simulink model "lab3_teil3fcn"  (R2018b)
settings: Solver=ode23t  StartTime=0.0  StopTime=10.0  RelTol=1e-12  AbsTol=1e-12
values from neighbouring files (symbols this model uses):
  AK = pi/4 * dK^2    (= 0.000314159265359)    [lab3_teil2.m]    (also in lab3_teil3.m; modelbildung_lab3.m)
  dB = 2.8e-3    (= 0.0028)    [lab3_teil2.m]    (also in lab3_teil3.m; modelbildung_lab3.m)
  FR = 5    [lab3_teil2.m]    (also in lab3_teil3.m; modelbildung_lab3.m)
  m = 1    [lab3_teil2.m]    (also in lab3_teil3.m; modelbildung_lab3.m)
  nB = table(:,2)    [lab3_teil3.m]
  rho = 850    [lab3_teil2.m]    (also in lab3_teil3.m; modelbildung_lab3.m)
  xB = table(:,1)    [lab3_teil3.m]
  zeta = 0.5    [lab3_teil2.m]    (also in lab3_teil3.m; modelbildung_lab3.m)
libraries: simulink x1
settings Model: Creator=Naveen  LastModifiedBy=Naveen

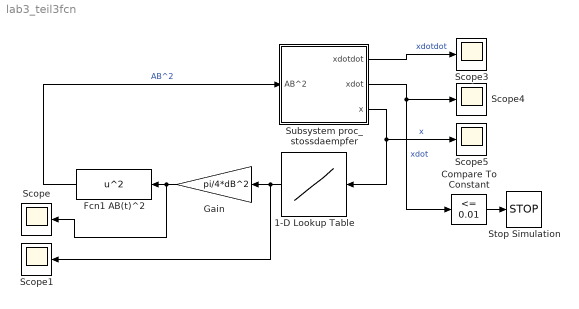
== system lab3_teil3fcn ==
  1-D Lookup Table : Lookup_n-D  NumberOfTableDimensions=1  BreakpointsForDimension1=xB  Table=nB  InternalRulePriority=Speed  RndMeth=Simplest  InputSameDT=on
  Compare To Constant : simulink/Logic and Bit Operations/Compare To Constant  relop=<=  const=0.01  OutDataTypeStr=boolean
  Fcn1 AB(t)^2 : Fcn  Expr=u^2
  Gain : Gain  Gain=pi/4*dB^2
  Scope{,1,3..5} (5 alike) : Scope
  Stop Simulation : Stop
  Subsystem proc_stossdaempfer : Subsystem
  wires:
  Subsystem proc_stossdaempfer/1(xdotdot) -> Scope3/1  "xdotdot"
  Subsystem proc_stossdaempfer/3(x) -> 1-D Lookup Table/1, Scope5/1  "x"
  Compare To Constant/1 -> Stop Simulation/1
  Subsystem proc_stossdaempfer/2(xdot) -> Compare To Constant/1, Scope4/1  "xdot"
  Fcn1 AB(t)^2/1 -> Subsystem proc_stossdaempfer/1(AB^2)  "AB^2"
  Gain/1 -> Scope/1, Fcn1 AB(t)^2/1
  1-D Lookup Table/1 -> Scope1/1, Gain/1

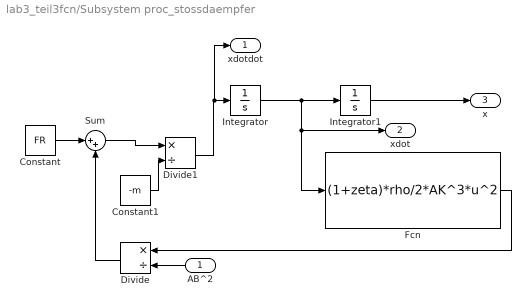
== system lab3_teil3fcn/Subsystem proc_stossdaempfer ==
  AB^2 : Inport
  Constant : Constant  Value=FR
  Constant1 : Constant  Value=-m
  Divide : Product  Inputs=*/
  Divide1 : Product  Inputs=*/
  Fcn : Fcn  Expr=(1+zeta)*rho/2*AK^3*u^2
  Integrator : Integrator  InitialCondition=3
  Integrator1 : Integrator  LimitOutput=on  LowerSaturationLimit=0
  Sum : Sum  Inputs=|++
  xdotdot : Outport
  xdot : Outport  Port=2
  x : Outport  Port=3
  wires:
  Integrator/1 -> Fcn/1, xdot/1, Integrator1/1
  Divide/1 -> Sum/2
  Constant1/1 -> Divide1/2
  Constant/1 -> Sum/1
  Divide1/1 -> xdotdot/1, Integrator/1
  Fcn/1 -> Divide/1
  Sum/1 -> Divide1/1
  Integrator1/1 -> x/1
  AB^2/1 -> Divide/2
